simulink model "sim_test"  (R2019a)
settings: Solver=FixedStepAuto  StartTime=0.0  StopTime=Inf  FixedStep=0.01  RelTol=1e-3
libraries: simulink x2, dspsigops x1, realtime_pacer_lib x1
settings Model: Creator=petter  LastModifiedBy=petter

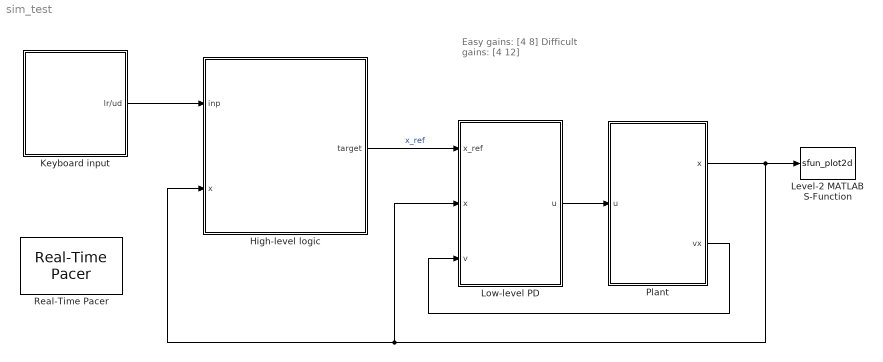
== system sim_test ==
  note: Easy gains:     [4 8]
      | Difficult gains: [4 12]
  High-level logic : Stateflow chart  BlockKeywords=__PRM__SERIALIZED__DATA__:Stateflow Chart,Stateflow Diagram  TreatAsAtomicUnit=on
  Keyboard input : Subsystem
  Level-2 MATLAB S-Function : M-S-Function  FunctionName=sfun_plot2d
  Low-level PD : Subsystem  mask{kx=4, kv=8}
  Plant : Subsystem  mask{x0=2.5, y0=2.5, a_max=2}
  Real-Time Pacer : realtime_pacer_lib/Real-Time Pacer  simTimePerRealTime=1
  wires:
  Plant/1(x) -> Low-level PD/2(x), High-level logic/2(x), Level-2 MATLAB S-Function/1
  High-level logic/1(target) -> Low-level PD/1(x_ref)  "x_ref"
  Plant/2(vx) -> Low-level PD/3(v)
  Low-level PD/1(u) -> Plant/1(u)
  Keyboard input/1(lr/ud) -> High-level logic/1(inp)

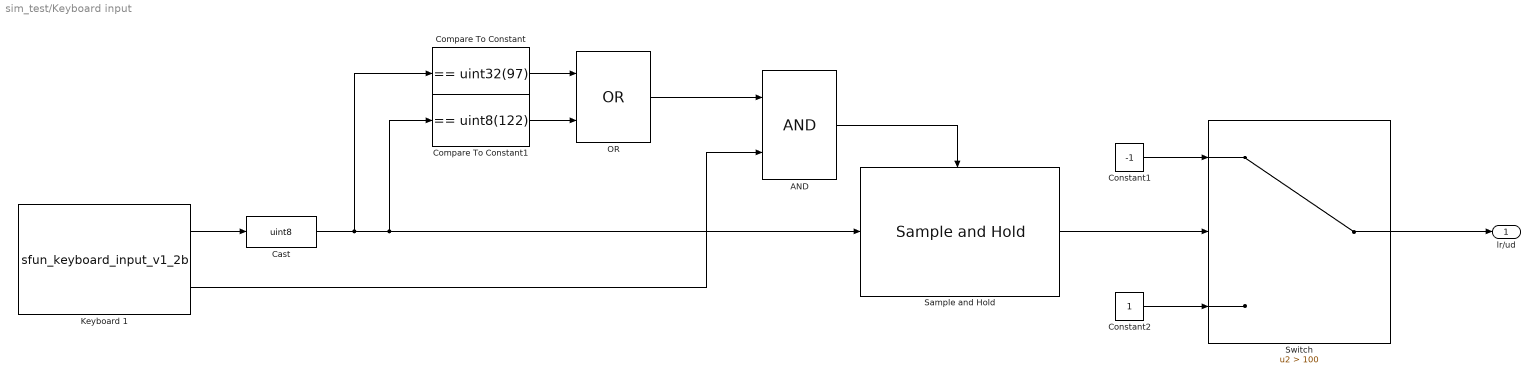
== system sim_test/Keyboard input ==
  AND : Logic  IconShape=distinctive  AllPortsSameDT=off  OutDataTypeStr=boolean
  Cast : DataTypeConversion  OutDataTypeStr=uint8
  Compare To Constant : simulink/Logic and Bit Operations/Compare To Constant  relop===  const=uint32(97)  OutDataTypeStr=boolean
  Compare To Constant1 : simulink/Logic and Bit Operations/Compare To Constant  relop===  const=uint8(122)  OutDataTypeStr=boolean
  Constant1 : Constant  Value=-1
  Constant2 : Constant
  Keyboard 1 : M-S-Function  FunctionName=sfun_keyboard_input_v1_2b  mask(Keyboard Input){}
      mask help: Keyboard Input
      mask Display: fprintf('Keyboard');
  OR : Logic  Operator=OR  IconShape=distinctive  AllPortsSameDT=off  OutDataTypeStr=boolean
  Sample and Hold : dspsigops/Sample and Hold  trig=Rising edge  initCond=97  latchinput=off
  Switch : Switch  Criteria=u2 > Threshold  Threshold=100
  lr/ud : Outport
  wires:
  Keyboard 1/1 -> Cast/1
  Compare To Constant/1 -> OR/1
  Constant1/1 -> Switch/1
  Switch/1 -> lr/ud/1
  Sample and Hold/1 -> Switch/2
  Compare To Constant1/1 -> OR/2
  Constant2/1 -> Switch/3
  Keyboard 1/2 -> AND/2
  Cast/1 -> Compare To Constant/1, Compare To Constant1/1, Sample and Hold/1
  OR/1 -> AND/1
  AND/1 -> Sample and Hold/Trigger

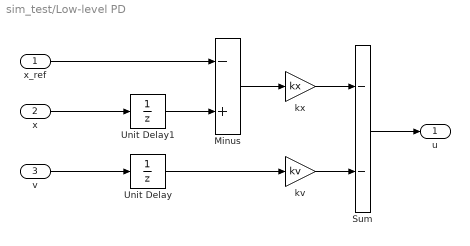
== system sim_test/Low-level PD ==
  x_ref : Inport
  x : Inport  Port=2
  v : Inport  Port=3
  Minus : Sum  Inputs=-+
  Sum : Sum  Inputs=--
  Unit Delay : UnitDelay  SampleTime=-1  HasFrameUpgradeWarning=on
  Unit Delay1 : UnitDelay  SampleTime=-1  HasFrameUpgradeWarning=on
  kv : Gain  Gain=kv
  kx : Gain  Gain=kx
  u : Outport
  wires:
  Unit Delay1/1 -> Minus/2
  kx/1 -> Sum/1
  kv/1 -> Sum/2
  x_ref/1 -> Minus/1
  x/1 -> Unit Delay1/1
  Minus/1 -> kx/1
  Unit Delay/1 -> kv/1
  Sum/1 -> u/1
  v/1 -> Unit Delay/1

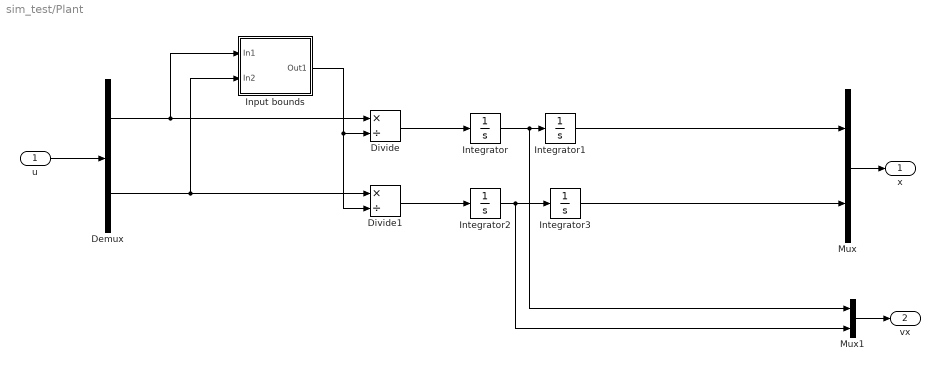
== system sim_test/Plant ==
  u : Inport
  Demux : Demux  Outputs=2
  Divide : Product  Inputs=*/
  Divide1 : Product  Inputs=*/
  Input bounds : Subsystem
  Integrator : Integrator
  Integrator1 : Integrator  InitialCondition=x0
  Integrator2 : Integrator
  Integrator3 : Integrator  InitialCondition=y0
  Mux : Mux  Inputs=2
  Mux1 : Mux  Inputs=2
  x : Outport
  vx : Outport  Port=2
  wires:
  Integrator1/1 -> Mux/1
  Integrator2/1 -> Mux1/2, Integrator3/1
  Integrator/1 -> Mux1/1, Integrator1/1
  Integrator3/1 -> Mux/2
  Divide/1 -> Integrator/1
  Divide1/1 -> Integrator2/1
  Input bounds/1(Out1) -> Divide1/2, Divide/2
  Demux/1 -> Divide/1, Input bounds/1(In1)
  Demux/2 -> Divide1/1, Input bounds/2(In2)
  u/1 -> Demux/1
  Mux/1 -> x/1
  Mux1/1 -> vx/1

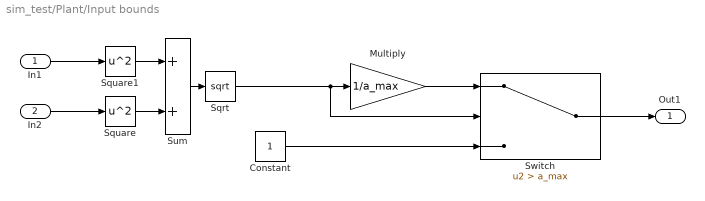
== system sim_test/Plant/Input bounds ==
  In1 : Inport
  In2 : Inport  Port=2
  Constant : Constant
  Multiply : Gain  Gain=1/a_max
  Sqrt : Sqrt  SaturateOnIntegerOverflow=on
  Square : Math  Operator=square  SaturateOnIntegerOverflow=on
  Square1 : Math  Operator=square  SaturateOnIntegerOverflow=on
  Sum : Sum
  Switch : Switch  Criteria=u2 > Threshold  Threshold=a_max
  Out1 : Outport
  wires:
  Multiply/1 -> Switch/1
  Switch/1 -> Out1/1
  In2/1 -> Square/1
  Constant/1 -> Switch/3
  In1/1 -> Square1/1
  Sqrt/1 -> Switch/2, Multiply/1
  Square/1 -> Sum/2
  Square1/1 -> Sum/1
  Sum/1 -> Sqrt/1

== stateflow chart sim_test/High-level logic ==
  state Top
    en:
    target = [2.5; 0.25];
    flag = -1;
  state Left
    en:
    flag = 1;
    target = [4.75; 2.5];
  state Center
    du:
    if inCenter(x)
    if inp < 0 && flag > 0
    target = [4.75; 2.5];
    elseif inp < 0 && flag < 0
    target = [0.25; 2.5];
    elseif inp > 0 && flag > 0
    target = [2.5; 4.75];
    elseif inp > 0 && flag < 0
    target = [2.5; 0.25];
    end
    end
  state Right
    en:
    target = [0.25; 2.5];
    flag = -1;
  state Bottom
    en:
    target = [2.5; 4.75];
    flag = 1;
  Top -> Center : [inCenter(x)]
  Center -> Top [order 1] : [x(2) > 4.25]
  (default) -> Center : {flag=1;}
  Right -> Center : [inCenter(x)]
  Center -> Left [order 4] : [x(1) < 0.75]
  Center -> Right [order 3] : [x(1) > 4.25]
  Left -> Center : [inCenter(x)]
  Center -> Bottom [order 2] : [x(2) < 0.75]
  Bottom -> Center : [inCenter(x)]
  data: inp input; x input; target output; flag local
